simulink model "WCDMA_Systems"  (R2021a)
settings: Solver=VariableStepAuto  StartTime=0.0  StopTime=10.0  RelTol=1e-3
settings Model: Creator=Ebenezer Sarpong  LastModifiedBy=Ebenezer Sarpong

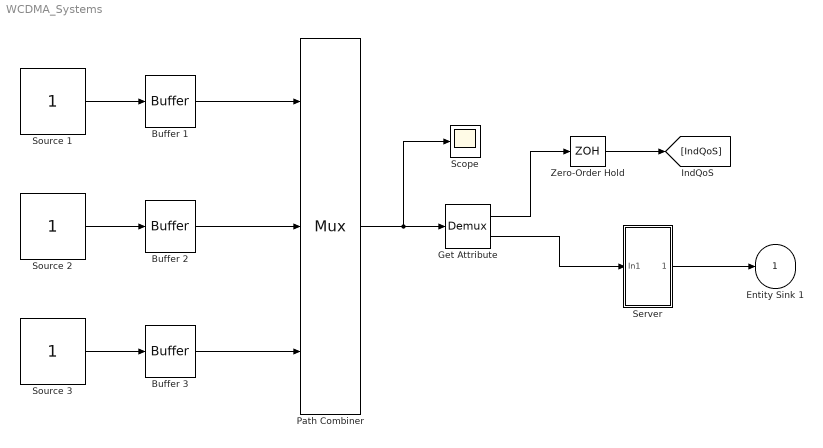
== system WCDMA_Systems ==
  Buffer 1 : Buffer  OutputFrames=off
  Buffer 2 : Buffer  N=65  OutputFrames=off
  Buffer 3 : Buffer  N=66  OutputFrames=off
  Get Attribute : Demux  Outputs=2
      settings: DisplayOption=none
  Path Combiner : Mux  Inputs=3
      settings: DisplayOption=signals
  Scope : Scope
  Server : Subsystem
  Source 1 : Constant
  Source 2 : Constant
  Source 3 : Constant
  Zero-Order Hold : ZeroOrderHold  SampleTime=-1
  Entity Sink 1 : Outport
  wires:
  Source 1/1 -> Buffer 1/1
  Source 2/1 -> Buffer 2/1
  Source 3/1 -> Buffer 3/1
  Buffer 1/1 -> Path Combiner/1
  Buffer 2/1 -> Path Combiner/2
  Buffer 3/1 -> Path Combiner/3
  Path Combiner/1 -> Scope/1, Get Attribute/1
  Get Attribute/2 -> Server/1(In1)
  Server/1(Entity Sink 1) -> Entity Sink 1/1
  Get Attribute/1 -> Zero-Order Hold/1
  Zero-Order Hold/1 -> [IndQoS]

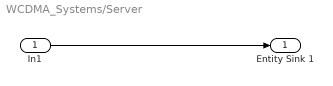
== system WCDMA_Systems/Server ==
  In1 : Inport
  Entity Sink 1 : Outport
  wires:
  In1/1 -> Entity Sink 1/1
